simulink model "modele5vBhrol"  (R2024a)
settings: Solver=VariableStepAuto  StartTime=0.0  StopTime=120  RelTol=1e-9
values from neighbouring files (symbols this model uses):
  A_L = 1    [etablissement_variables.m]
  A_S = 3    [etablissement_variables.m]
  C_x = 0.2    [etablissement_variables.m]
  Cte_1 = 10    [etablissement_variables.m]
  Cte_2 = 1.9    [etablissement_variables.m]
  Cte_3 = 1    [etablissement_variables.m]
  Cte_4 = 0.97    [etablissement_variables.m]
  d_f = 1    [etablissement_variables.m]
  d_r = 1    [etablissement_variables.m]
  EPSILON = 1e-9    (= 1e-09)    [etablissement_variables.m]
  f = 0.1    [etablissement_variables.m]
  g = 9.81    [etablissement_variables.m]
  h = 0.4    [etablissement_variables.m]
  Iz = 500    [etablissement_variables.m]
  J = mr/2*R.^2    [etablissement_variables.m]
  L = l_r+l_f    (= 2.9)    [etablissement_variables.m]
  l_f = 1.7    [etablissement_variables.m]
  l_r = 1.2    [etablissement_variables.m]
  M = 400    [etablissement_variables.m]
  R = [0.52 0.52 0.52 0.52]    [etablissement_variables.m]
  rho = 1    [etablissement_variables.m]
undefined symbols (not defined in the file or in its folder): calcul_adherence, calcul_delta, calcul_forceaero, calcul_forces, calcul_lambda, calcul_moteur, calcul_N, calcul_normevitesseroue, calcul_omega, calcul_omegaackermann, calcul_retourvitesse, calcul_rotaroute, calcul_slipangle, calcul_vitessesroues, check_zeros_1, check_zeros_8, eqpfd, projection, reconstructionPi
libraries: simulink x5, slpidlib x2, embmathops x1
settings Model: Creator=TP-EEA  LastModifiedBy=TP-EEA

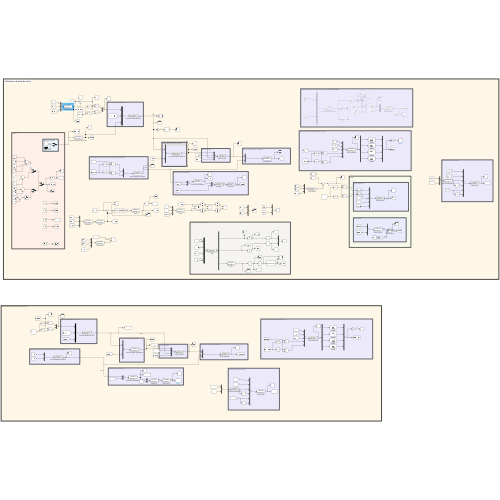
[thumbnail: Simulink's stored preview of the top-level diagram]
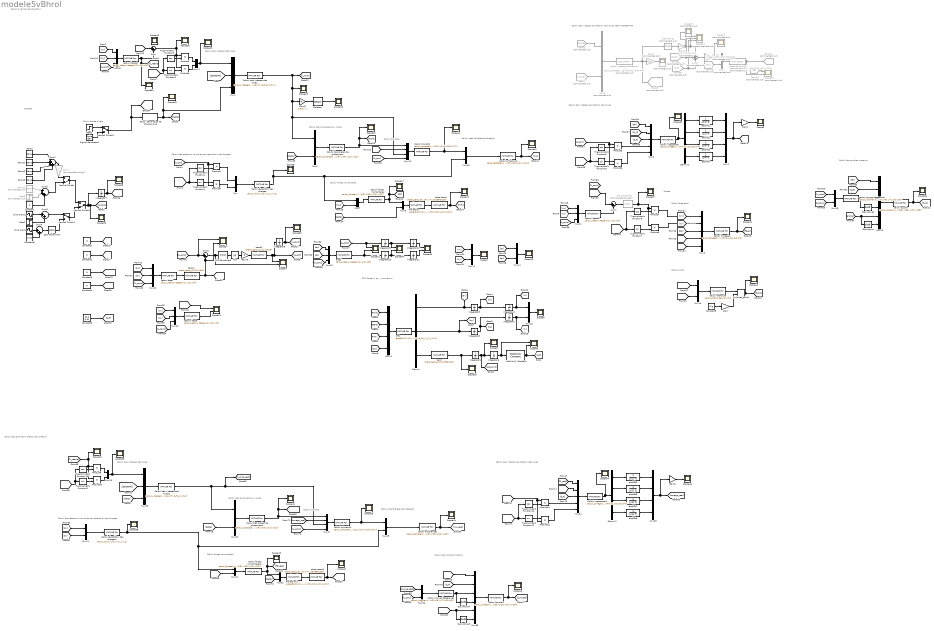
== system modele5vBhrol ==
  note: Calcul des grandeurs réelles (sans retour)
  note: Calcul avec boucle de retour
  note: Calcul des vitesses des roues
  note: Entrées
  note: Choix entrée angle
  note: Calcul des vitesses de rotation des roues
  note: PFD (forces x et y, moment z)
  note: Calcul poids
  note: Calcul des slip-angle aux roues
  note: Calcul coef adhérence (Pacejka)
  note: Calcul slip-ratio
  note: Calcul des réactions normales par répartition des charges
  note: Calcul forces horizontales
  note: Forces
  note: Calcul force aéro
  note: Calcul des vitesses de rotation des roues TEST ACKERMANN
  note: Calcul des réactions normales par répartition des charges
  note: Calcul des couples moteurs
  note: Calcul des vitesses des roues
  note: Calcul slip-ratio
  note: Calcul coef adhérence (Pacejka)
  note: Calcul des slip-angle aux roues
  note: Calcul forces horizontales
  note: Calcul des vitesses de rotation des roues
  note: Calcul des couples moteurs
  Abs : Abs  SaturateOnIntegerOverflow=off
  Calcul adhérence : MATLABFcn  MATLABFcn=calcul_adherence(u(1),u(2),u(3),u(4),u(5),u(6),u(7),u(8),Cte_1,Cte_2,Cte_3,Cte_4,u(9),u(10),u(11),u(12))  OutputDimensions=4*2
  Calcul adhérence1 : MATLABFcn  MATLABFcn=calcul_adherence(u(1),u(2),u(3),u(4),u(5),u(6),u(7),u(8),Cte_1,Cte_2,Cte_3,Cte_4,u(9),u(10),u(11),u(12))  OutputDimensions=4*2
  Calcul des angles de chaque roue : MATLABFcn  MATLABFcn=calcul_delta(u,L,d_f)  OutputDimensions=4
  Calcul des angles de glissement : MATLABFcn  MATLABFcn=calcul_slipangle(u(1),u(2),u(3),u(4),u(5),u(6),u(7),u(8),u(9),u(10),u(11),u(12))  OutputDimensions=4
  Calcul des angles de glissement1 : MATLABFcn  MATLABFcn=calcul_slipangle(u(1),u(2),u(3),u(4),u(5),u(6),u(7),u(8),u(9),u(10),u(11),u(12))  OutputDimensions=4
  Calcul des vitesses des roues : MATLABFcn  MATLABFcn=calcul_vitessesroues(u(1),u(2),u(3),u(4),u(5),u(6),u(7),d_f,d_r,l_f,l_r)  OutputDimensions=8
  Calcul des vitesses des roues1 : MATLABFcn  MATLABFcn=calcul_vitessesroues(u(1),u(2),u(3),u(4),u(5),u(6),u(7),d_f,d_r,l_f,l_r)  OutputDimensions=8
  Calcul forceaéro : MATLABFcn  MATLABFcn=calcul_forceaero(u(1),u(2),u(3),u(4),u(5),C_x,A_L,A_S,rho)  OutputDimensions=2
  Calcul forces horizontales : MATLABFcn  MATLABFcn=calcul_forces(u(1),u(2),u(3),u(4),u(5),u(6),u(7),u(8),u(9),u(10),u(11),u(12))  OutputDimensions=4*2
  Calcul forces horizontales1 : MATLABFcn  MATLABFcn=calcul_forces(u(1),u(2),u(3),u(4),u(5),u(6),u(7),u(8),u(9),u(10),u(11),u(12))  OutputDimensions=4*2
  Calcul rotaroute : MATLABFcn  MATLABFcn=calcul_rotaroute(u(1),u(2))  OutputDimensions=[3 3]  Output1D=off
  Calcul répartition des charges : MATLABFcn  MATLABFcn=calcul_N(u(1),u(2),M,L,l_r,h,g)  OutputDimensions=4
  Calcul répartition des charges1 : MATLABFcn  MATLABFcn=calcul_N(u(1),u(2),M,L,l_r,h,g)  OutputDimensions=4
  Calcul slip-ratio : MATLABFcn  MATLABFcn=calcul_lambda(u(1),u(2),u(3),u(4),R(1),R(2),R(3),R(4),u(5),u(6),u(7),u(8),u(9),u(11),u(13),u(15),u(10),u(12),u(14),u(16),u(17))  OutputDimensions=4*2
  Calcul slip-ratio1 : MATLABFcn  MATLABFcn=calcul_lambda(u(1),u(2),u(3),u(4),R(1),R(2),R(3),R(4),u(5),u(6),u(7),u(8),u(9),u(11),u(13),u(15),u(10),u(12),u(14),u(16),u(17))  OutputDimensions=4*2
  Calcul vitesserota : MATLABFcn  MATLABFcn=calcul_omega(u(1),u(2),u(3),u(4),u(5),u(6),u(7),u(8),u(9),u(10),u(11),u(12),u(13),u(14),u(15),u(16),u(17),u(18),R(1),R(2),R(3),R(4),J(1),J(2),J(3),J(4))  OutputDimensions=4
  Calcul vitesserota1 : MATLABFcn  MATLABFcn=calcul_omega(u(1),u(2),u(3),u(4),u(5),u(6),u(7),u(8),u(9),u(10),u(11),u(12),u(13),u(14),u(15),u(16),u(17),u(18),R(1),R(2),R(3),R(4),J(1),J(2),J(3),J(4))  OutputDimensions=4
  Calcul vitesserotaAckermann : MATLABFcn  Commented=on  MATLABFcn=calcul_omegaackermann(u(1),u(2),u(3),u(4),u(5),u(6),u(7),u(8),u(9),u(10),u(11),u(12),R(1),R(2),R(3),R(4))  OutputDimensions=4
  Constant{,1..4} (5 alike) : Constant  Value=0
  Constant5 : Constant  Value=M*g  VectorParams1D=off
  Constant6 : Constant  Value=1.01
  Constant8 : Constant  Value=[0 0 0 0]
  Demux : Demux  Outputs=3
  Demux1 : Demux
  Demux2 : Demux
  Derivative{,2..4} (4 alike) : Derivative
  Derivative1 : Derivative  Commented=on
  From12 : From  Commented=on  GotoTag=V_roue
  From36 : From  Commented=on  GotoTag=C_M
  From39 : From  Commented=on  GotoTag=C_F
  From43 : From  Commented=on  GotoTag=FP
  From46 : From  Commented=on  GotoTag=mu
  From6 : From  Commented=on  GotoTag=alpha
  Gain : Gain  Gain=[0 0 1]'
  Gain1 : Gain  Gain=30/pi
  Gain2 : Gain  Commented=on  Gain=[J(1) J(2) J(3) J(4)]
  Gain3 : Gain  Commented=on  Gain=-1./[R(1) R(2) R(3) R(4)]
  Gain4 : Gain  Commented=on  Gain=30/pi
  Gain5 : Gain  Gain=1/R(1)  Multiplication=Matrix(K*u)
  Gain6 : Gain  Gain=30/pi
  Gain7 : Gain  Commented=through  Gain=-1  Multiplication=Matrix(K*u)
  Gain8 : Gain  Gain=-1
  Goto24 : Goto  Commented=on  GotoTag=Fi_comp
  Goto25 : Goto  Commented=on  GotoTag=omega_comp
  Integrator{1..12} (12 alike) : Integrator
  Manual Switch : ManualSwitch  CurrentSetting=0
  Manual Switch1 : ManualSwitch
  Manual Switch2 : ManualSwitch
  Manual Switch3 : ManualSwitch  CurrentSetting=0
  Modulo by Constant : embmathops/Modulo by Constant  Denominator=2*pi  SimulateUsing=Code generation
      settings: LibrarySourceBlock=embeddedMathLib/Modulo by Constant
  Mux{,6..8,10,12..14,16..17,24..26,29..32,36} (18 alike) : Mux  Inputs=2
  Mux{1,11,15,27,33} (5 alike) : Mux
  Mux{2,18..22,28} (7 alike) : Mux  Inputs=3
  Mux23 : Mux  Inputs=6
  Mux3 : Mux  Commented=on  Inputs=2
  Mux34 : Mux  Inputs=5
  Mux35 : Mux  Inputs=6
  Mux4 : Mux  Commented=on  Inputs=2
  Mux5 : Mux  Inputs=5
  Mux9 : Mux  Inputs=5
  PFD : MATLABFcn  MATLABFcn=eqpfd(u(1),u(2),u(4),u(5),u(6),u(7),u(8),u(9),u(10),u(11),u(12),u(13),u(14),d_f,d_r,l_f,l_r,M,Iz)  OutputDimensions=3
  PID Controller1 : slpidlib/PID Controller  Commented=through  Controller=PID  Form=Parallel  TimeDomain=Continuous-time  UseExternalTs=off  SampleTime=-1  IntegratorMethod=Forward Euler  FilterMethod=Forward Euler  ControllerParametersSource=internal  P=5  I=1  UseKiTs=off  D=10  UseExternalDerivativeSource=off  N=100  UseFilter=on  TunerSelectOption=Transfer Function Based (PID Tuner App)  InitialConditionSource=internal  InitialConditionForIntegrator=0  InitialConditionForFilter=0  DifferentiatorICPrevScaledInput=0  ExternalReset=none  TrackingMode=off  Kt=1  LimitOutput=off  SatLimitsSource=internal  UpperSaturationLimit=inf  LowerSaturationLimit=-inf  LinearizeAsGain=on  AntiWindupMode=none  Kb=1  LimitIntegrator=off  UpperIntegratorSaturationLimit=inf  LowerIntegratorSaturationLimit=-inf  POutMin=[]  POutMax=[]  IOutMin=[]  IOutMax=[]  DOutMin=[]  DOutMax=[]  NOutMin=[]  NOutMax=[]  SumOutMin=[]  SumOutMax=[]  SaturationOutMin=[]  SaturationOutMax=[]  PParamMin=[]  PParamMax=[]  IParamMin=[]  IParamMax=[]  DParamMin=[]  DParamMax=[]  NParamMin=[]  NParamMax=[]  KbParamMin=[]  KbParamMax=[]  KtParamMin=[]  KtParamMax=[]  KbOutMin=[]  KbOutMax=[]  KtOutMin=[]  KtOutMax=[]  IntegratorOutMin=[]  IntegratorOutMax=[]  FilterOutMin=[]  FilterOutMax=[]  SumI1OutMin=[]  SumI1OutMax=[]  SumI2OutMin=[]  SumI2OutMax=[]  SumI3OutMin=[]  SumI3OutMax=[]  SumI4OutMin=[]  SumI4OutMax=[]  SumDOutMin=[]  SumDOutMax=[]  DifferentiatorOutMin=[]  DifferentiatorOutMax=[]  FilterDiffOutCoefMin=[]  FilterDiffOutCoefMax=[]  ReciprocalOutMin=[]  ReciprocalOutMax=[]  SumDenOutMin=[]  SumDenOutMax=[]  SumNumOutMin=[]  SumNumOutMax=[]  DivideOutMin=[]  DivideOutMax=[]  UdiffTsProdOutMin=[]  UdiffTsProdOutMax=[]  NTsProdOutMin=[]  NTsProdOutMax=[]  UintegralTsProdOutMin=[]  UintegralTsProdOutMax=[]  UngainTsProdOutMin=[]  UngainTsProdOutMax=[]  ClampingZeroOutDataTypeStr=Inherit: Inherit via back propagation  ClampingZeroOutMin=[]  ClampingZeroOutMax=[]  FilterDenConstantOutDataTypeStr=Inherit: Inherit via back propagation  FilterDenConstantOutMin=[]  FilterDenConstantOutMax=[]  PCopyOutDataTypeStr=Inherit: Inherit via back propagation  PCopyOutMin=[]  PCopyOutMax=[]  NCopyOutDataTypeStr=Inherit: Inherit via back propagation  NCopyOutMin=[]  NCopyOutMax=[]  IntegratorContinuousStateAttributes=''  IntegratorStateMustResolveToSignalObject=off  IntegratorRTWStateStorageClass=Auto  FilterContinuousStateAttributes=''  FilterStateMustResolveToSignalObject=off  FilterRTWStateStorageClass=Auto  ParallelPVariant=InternalParameters  IdealPVariant=Disabled  IVariant=InternalParameters  DVariant=InternalParameters  IntegratorVariant=Continuous  SatVariant=Disabled  AWVariant=Passthrough  PCopyVariant=Disabled  TRVariant=Disabled  FdbkBlocksVariant=Forward  IdealPFdbkVariant=Disabled  SatFdbkVariant=Disabled  DerivativeFilterVariant=ContFilter  NVariant=InternalParameters  NCopyVariant=Disabled  FilterICVariant=InternalICsFilter  IntegratorICVariant=InternalICs  ExternalResetVariant=Disabled  TRSumVariant=Passthrough  SumFdbkVariant=Disabled  SumVariant=Sum_PID  TsampFilterVariant=InternalTs  TsampNgainVariant=Passthrough  TsampIntegralVariant=Disabled_SignalSpec  ExternalSaturationOutDataTypeStr=Inherit: Same as second input  DerivativeSourceVariant=ErrorSignal
  PID Controller3 : slpidlib/PID Controller  Controller=PID  Form=Ideal  TimeDomain=Continuous-time  UseExternalTs=off  SampleTime=-1  IntegratorMethod=Forward Euler  FilterMethod=Forward Euler  ControllerParametersSource=internal  P=1  I=100  UseKiTs=off  D=0  UseExternalDerivativeSource=off  N=300  UseFilter=on  TunerSelectOption=Frequency Response Based  InitialConditionSource=internal  InitialConditionForIntegrator=0  InitialConditionForFilter=0  DifferentiatorICPrevScaledInput=0  ExternalReset=none  TrackingMode=off  Kt=1  LimitOutput=off  SatLimitsSource=internal  UpperSaturationLimit=inf  LowerSaturationLimit=-inf  LinearizeAsGain=on  AntiWindupMode=none  Kb=1  LimitIntegrator=off  UpperIntegratorSaturationLimit=inf  LowerIntegratorSaturationLimit=-inf  POutMin=[]  POutMax=[]  IOutMin=[]  IOutMax=[]  DOutMin=[]  DOutMax=[]  NOutMin=[]  NOutMax=[]  SumOutMin=[]  SumOutMax=[]  SaturationOutMin=[]  SaturationOutMax=[]  PParamMin=[]  PParamMax=[]  IParamMin=[]  IParamMax=[]  DParamMin=[]  DParamMax=[]  NParamMin=[]  NParamMax=[]  KbParamMin=[]  KbParamMax=[]  KtParamMin=[]  KtParamMax=[]  KbOutMin=[]  KbOutMax=[]  KtOutMin=[]  KtOutMax=[]  IntegratorOutMin=[]  IntegratorOutMax=[]  FilterOutMin=[]  FilterOutMax=[]  SumI1OutMin=[]  SumI1OutMax=[]  SumI2OutMin=[]  SumI2OutMax=[]  SumI3OutMin=[]  SumI3OutMax=[]  SumI4OutMin=[]  SumI4OutMax=[]  SumDOutMin=[]  SumDOutMax=[]  DifferentiatorOutMin=[]  DifferentiatorOutMax=[]  FilterDiffOutCoefMin=[]  FilterDiffOutCoefMax=[]  ReciprocalOutMin=[]  ReciprocalOutMax=[]  SumDenOutMin=[]  SumDenOutMax=[]  SumNumOutMin=[]  SumNumOutMax=[]  DivideOutMin=[]  DivideOutMax=[]  UdiffTsProdOutMin=[]  UdiffTsProdOutMax=[]  NTsProdOutMin=[]  NTsProdOutMax=[]  UintegralTsProdOutMin=[]  UintegralTsProdOutMax=[]  UngainTsProdOutMin=[]  UngainTsProdOutMax=[]  ClampingZeroOutDataTypeStr=Inherit: Inherit via back propagation  ClampingZeroOutMin=[]  ClampingZeroOutMax=[]  FilterDenConstantOutDataTypeStr=Inherit: Inherit via back propagation  FilterDenConstantOutMin=[]  FilterDenConstantOutMax=[]  PCopyOutDataTypeStr=Inherit: Inherit via back propagation  PCopyOutMin=[]  PCopyOutMax=[]  NCopyOutDataTypeStr=Inherit: Inherit via back propagation  NCopyOutMin=[]  NCopyOutMax=[]  IntegratorContinuousStateAttributes=''  IntegratorStateMustResolveToSignalObject=off  IntegratorRTWStateStorageClass=Auto  FilterContinuousStateAttributes=''  FilterStateMustResolveToSignalObject=off  FilterRTWStateStorageClass=Auto  ParallelPVariant=Passthrough  IdealPVariant=InternalParameters  IVariant=InternalParameters  DVariant=InternalParameters  IntegratorVariant=Continuous  SatVariant=Disabled  AWVariant=Passthrough  PCopyVariant=Disabled  TRVariant=Disabled  FdbkBlocksVariant=Forward  IdealPFdbkVariant=Disabled  SatFdbkVariant=Disabled  DerivativeFilterVariant=ContFilter  NVariant=InternalParameters  NCopyVariant=Disabled  FilterICVariant=InternalICsFilter  IntegratorICVariant=InternalICs  ExternalResetVariant=Disabled  TRSumVariant=Passthrough  SumFdbkVariant=Disabled  SumVariant=Sum_PID  TsampFilterVariant=InternalTs  TsampNgainVariant=Passthrough  TsampIntegralVariant=Disabled_SignalSpec  ExternalSaturationOutDataTypeStr=Inherit: Same as second input  DerivativeSourceVariant=ErrorSignal
  Product{1..12} (12 alike) : Product
  Projection : MATLABFcn  MATLABFcn=projection(u(1),u(2),u(3),u(4),u(5),u(6),u(7),u(8),u(9),u(10),u(11),u(12))  OutputDimensions=8
  Projection1 : MATLABFcn  MATLABFcn=projection(u(1),u(2),u(3),u(4),u(5),u(6),u(7),u(8),u(9),u(10),u(11),u(12))  OutputDimensions=8
  Ramp : simulink/Sources/Ramp  slope=1  start=0  InitialOutput=0
  Ramp1 : simulink/Sources/Ramp  slope=-1  start=3  InitialOutput=0
  Ramp2 : simulink/Sources/Ramp  slope=-1  start=7  InitialOutput=0
  Ramp3 : simulink/Sources/Ramp  slope=1  start=9  InitialOutput=0
  Ramp4 : simulink/Sources/Ramp  Commented=on  slope=-1  start=0  InitialOutput=0
  ReconstructionPi : MATLABFcn  Commented=on  MATLABFcn=reconstructionPi(u(1),u(2),u(3),u(4),u(5),u(6),u(7),u(8),u(9),u(10),u(11),u(12))  OutputDimensions=8
  Scope1 : Scope  Commented=on
  Scope{2..3,6..8,10..20,25..26,28..30,32..33,36..50} (38 alike) : Scope
  Scope{4,9,21..22,27,34..35} (7 alike) : Scope  NumInputPorts=2
  Scope23 : Scope  Commented=on  NumInputPorts=2
  Scope24 : Scope  Commented=on  NumInputPorts=3
  Scope31 : Scope  Commented=on
  Scope5 : Scope  Commented=on
  Selector : Selector  InputPortWidth=8  IndexOptions=Index vector (dialog)  Indices=[1,3,5,7]  OutputSizes=1
  Signal Generator2 : SignalGenerator  Amplitude=0.2  Frequency=0.1  Units=rad/sec
  Sine Wave : Sin  Frequency=0.1  SampleTime=0
  Sine Wave1 : Sin  SampleTime=0
  Step1 : Step  Time=0  After=0  SampleTime=0
  Step2 : Step  Time=0  After=0  SampleTime=0
  Step3 : Step  Commented=on  Time=0  SampleTime=0
  Sum : Sum  Inputs=|+-
  Sum1 : Sum  Inputs=|++++
  Sum2 : Sum  Commented=on  Inputs=+-+
  Sum3 : Sum  Inputs=|+-
  Sum4 : Sum  Inputs=|++
  Sum5 : Sum  Inputs=|++
  Sum6 : Sum  Inputs=|+++
  Sum7 : Sum  Inputs=|+-
  Trigonometric Function{1..2,5,7,9,11} (6 alike) : Trigonometry
  Trigonometric Function{3..4,6,8,10,12} (6 alike) : Trigonometry  Operator=cos
  Zero-Order Hold : ZeroOrderHold  SampleTime=3
  accel : MATLABFcn  MATLABFcn=calcul_retourvitesse(u(1),u(2),u(3))  OutputDimensions=1
  calcul couple : MATLABFcn  MATLABFcn=calcul_moteur(u(1),u(2),u(3),u(4),u(5),u(6),u(7),u(8),u(9),u(10),u(11),u(12),R(1),R(2),R(3),R(4),J(1),J(2),J(3),J(4),u(13),u(14),u(15),u(16),u(17),u(18),u(19),u(20),u(21),u(22),u(23),u(24),u(25),u(26),u(27),u(28))  OutputDimensions=4
  calcul couple1 : MATLABFcn  MATLABFcn=calcul_moteur(u(1),u(2),u(3),u(4),u(5),u(6),u(7),u(8),u(9),u(10),u(11),u(12),R(1),R(2),R(3),R(4),J(1),J(2),J(3),J(4),u(13),u(14),u(15),u(16),u(17),u(18),u(19),u(20),u(21),u(22),u(23),u(24),u(25),u(26),u(27),u(28))  OutputDimensions=4
  calcul normevitesseroue : MATLABFcn  MATLABFcn=calcul_normevitesseroue(u(1),u(2),u(3),u(4),u(5),u(6),u(7),u(8),u(9))  OutputDimensions=4
  calcul normevitesseroue1 : MATLABFcn  MATLABFcn=calcul_normevitesseroue(u(1),u(2),u(3),u(4),u(5),u(6),u(7),u(8),u(9))  OutputDimensions=4
  check zeros : MATLABFcn  MATLABFcn=check_zeros_8(u(1),u(2),u(3),u(4),u(5),u(6),u(7),u(8),EPSILON)  OutputDimensions=8
  check zeros1 : MATLABFcn  MATLABFcn=check_zeros_8(u(1),u(2),u(3),u(4),u(5),u(6),u(7),u(8),EPSILON)  OutputDimensions=8
  eqdiffz1 : TransferFcn  Denominator=[J(1) f]
  eqdiffz2 : TransferFcn  Denominator=[J(2) f]
  eqdiffz3 : TransferFcn  Denominator=[J(3) f]
  eqdiffz4 : TransferFcn  Denominator=[J(4) f]
  eqdiffz5 : TransferFcn  Denominator=[J(1) f]
  eqdiffz6 : TransferFcn  Denominator=[J(2) f]
  eqdiffz7 : TransferFcn  Denominator=[J(3) f]
  eqdiffz8 : TransferFcn  Denominator=[J(4) f]
  multmat_poids : Product  Multiplication=Matrix(*)
  retour accel : MATLABFcn  MATLABFcn=calcul_retourvitesse(u(1),u(2),u(3))  OutputDimensions=1
  retourvitesse : MATLABFcn  MATLABFcn=calcul_retourvitesse(u(1),u(2),u(3))  OutputDimensions=1
  retourvitesse1 : MATLABFcn  MATLABFcn=calcul_retourvitesse(u(1),u(2),u(3))  OutputDimensions=1
  retourvitesse2 : MATLABFcn  MATLABFcn=calcul_retourvitesse(u(1),u(2),u(3))  OutputDimensions=1
  zeros : MATLABFcn  MATLABFcn=check_zeros_1(u(1),EPSILON)
  zeros1 : MATLABFcn  MATLABFcn=check_zeros_1(u(1),1e-9)
  zeros2 : MATLABFcn  MATLABFcn=check_zeros_1(u(1),1e-15)
  wires:
  accel/1 -> Integrator10/1, Scope21/2
  Calcul des angles de glissement/1 -> [alpha], Scope13/1, Mux15/1
  Mux17/1 -> Scope20/1, Mux2/1
  [Vventy] -> Mux9/5
  [ay] -> Mux22/2
  [ax] -> Mux22/1
  Mux9/1 -> Calcul forceaéro/1
  Mux2/1 -> Calcul des vitesses des roues/1
  Calcul adhérence/1 -> Scope16/1, [mu]
  [A_cons] -> Scope27/1, Sum3/1
  Mux22/1 -> retour accel/1
  [thetaroute] -> Mux10/1
  [Vx] -> Mux20/1
  eqdiffz4/1 -> Mux1/4
  [Faero] -> Mux11/2
  retourvitesse/1 -> Scope22/2  "V"
  [ax] -> Mux19/1
  Mux11/1 -> PFD/1
  [A_cons] -> Integrator9/1, Scope21/1
  [Poids] -> Mux11/1
  Manual Switch2/1 -> [delta_com], Calcul des angles de chaque roue/1
  Trigonometric Function3/1 -> Product2/2
  Product2/1 -> Mux17/1
  Projection/1 -> check zeros/1  "FxFy"
  Trigonometric Function2/1 -> Product3/2
  [A_corr] -> Mux15/4
  PFD/1 -> Demux/1
  Mux8/1 -> Projection/1
  Constant5/1 -> Gain/1
  Mux6/1 -> Calcul des angles de glissement/1
  Integrator2/1 -> Mux13/2, [y]
  Mux7/1 -> Calcul forces horizontales/1
  multmat_poids/1 -> Scope11/1, [Poids]  "P"
  Product3/1 -> Mux17/2
  Mux10/1 -> Calcul rotaroute/1
  Calcul forceaéro/1 -> Scope10/1, [Faero]  "forceaéro"
  Integrator1/1 -> Scope8/1, Integrator6/1, [psipoint]
  Mux15/1 -> Calcul slip-ratio/1
  [FxFy] -> Mux11/3
  [delta_com] -> Trigonometric Function3/1, Trigonometric Function2/1
  Gain/1 -> multmat_poids/2
  Mux20/1 -> retourvitesse/1
  [mu] -> Mux7/2
  Mux14/1 -> Scope15/1
  [psipoint] -> Mux2/2
  Integrator4/1 -> Mux13/1, [x]
  [Vventx] -> Mux9/4
  [psi] -> Mux9/3
  [ax] -> Mux14/1
  [ay] -> Mux14/2
  Mux12/1 -> Scope7/1
  Integrator5/1 -> Integrator4/1, [Vx]
  [phiroute] -> Mux10/2
  Integrator6/1 -> Modulo by Constant/1, Scope9/1
  [Vx] -> Mux12/1
  Mux13/1 -> Scope3/1
  Signal Generator2/1 -> Manual Switch2/2  "delta*"
  eqdiffz3/1 -> Mux1/3
  calcul couple/1 -> Scope36/1, [C_M]
  [Vy] -> Mux12/2
  Step1/1 -> Manual Switch2/1  "delta*"
  Calcul rotaroute/1 -> multmat_poids/1
  Constant1/1 -> [Vventx]
  Calcul des angles de chaque roue/1 -> [delta], Mux2/3, Scope18/1
  Calcul répartition des charges/1 -> Mux7/1, Mux16/2, Scope6/1  "N_cons"
  Constant4/1 -> [phiroute]
  Constant2/1 -> [Vventy]
  Integrator3/1 -> Integrator2/1, [Vy]
  Demux1/4 -> eqdiffz4/1
  Constant8/1 -> [C_F]
  eqdiffz2/1 -> Mux1/2
  [C_M] -> Mux5/2
  Mux19/1 -> accel/1
  Mux5/1 -> Calcul vitesserota/1
  Calcul vitesserota/1 -> Scope32/1, Demux1/1
  [delta] -> Mux8/2
  retour accel/1 -> zeros1/1  "A_ret"
  Mux1/1 -> Gain1/1, [omega]
  [C_F] -> Mux5/3
  eqdiffz1/1 -> Mux1/1
  Constant3/1 -> [thetaroute]
  Demux1/3 -> eqdiffz3/1
  Demux1/2 -> eqdiffz2/1
  Demux1/1 -> eqdiffz1/1
  Product4/1 -> Mux/2
  [ay] -> Mux19/2
  [Vy] -> Mux20/2
  Modulo by Constant/1 -> [psi], Scope9/2
  Manual Switch3/1 -> Integrator7/1, Scope33/1, [A_cons]
  Manual Switch/1 -> Manual Switch3/1
  Manual Switch1/1 -> Manual Switch3/2
  Zero-Order Hold/1 -> Manual Switch1/2
  Gain1/1 -> Scope2/1
  Sum1/1 -> Gain7/1
  From12/1 -> Mux3/2
  Mux3/1 -> Calcul vitesserotaAckermann/1
  Calcul vitesserotaAckermann/1 -> Gain4/1, Derivative1/1, Goto25/1
  Derivative1/1 -> Gain2/1
  Gain2/1 -> Scope31/1, Scope24/1, Sum2/1
  From36/1 -> Scope24/2, Sum2/2
  From39/1 -> Scope24/3, Sum2/3
  Sum2/1 -> Gain3/1
  From43/1 -> Scope23/1
  [omega] -> Mux15/2
  From46/1 -> Mux4/2
  Gain3/1 -> Scope1/1, Mux4/1
  Mux4/1 -> ReconstructionPi/1
  ReconstructionPi/1 -> Goto24/1, Scope23/2
  [FP] -> Mux5/1
  [V_voulue] -> Scope22/1  "Vvoulue"
  zeros/1 -> Scope29/1, Integrator1/1
  Gain4/1 -> Scope5/1
  Integrator8/1 -> Scope30/1, [V_cons]
  PID Controller3/1 -> Abs/1
  Gain5/1 -> Selector/1
  Selector/1 -> Scope25/1
  From6/1 -> Mux3/1
  [Vy] -> Mux18/2
  [Vx] -> Mux18/1
  [V_voulue] -> Sum/1
  retourvitesse2/1 -> Sum/2, Scope50/1, [V_reelle]  "V"
  Mux18/1 -> retourvitesse2/1
  [psi] -> Mux11/4
  [delta] -> Mux6/2
  Calcul forces horizontales/1 -> Scope17/1, [FP], Mux8/1
  Mux/1 -> Calcul répartition des charges/1
  Calcul des vitesses des roues/1 -> Gain5/1, Mux6/1, Mux15/3, Scope19/1, [V_roue]  "Vrcons"
  [FP] -> Mux23/1
  [C_F] -> Mux23/2
  Mux23/1 -> calcul couple/1
  check zeros/1 -> Scope12/1, [FxFy]  "FxFy"
  Sum/1 -> Scope26/1, Product3/1, Product2/1
  Ramp/1 -> Sum1/1
  Ramp1/1 -> Sum1/2
  Ramp2/1 -> Sum1/3
  Ramp3/1 -> Sum1/4
  Integrator7/1 -> [V_voulue], Scope28/1
  [delta_com] -> Trigonometric Function4/1, Trigonometric Function1/1
  Trigonometric Function1/1 -> Product4/1
  Product1/1 -> Mux/1
  Trigonometric Function4/1 -> Product1/2
  [A_corr] -> Product1/1, Product4/2
  Product5/1 -> Mux5/4
  [delta_com] -> Trigonometric Function6/1, Trigonometric Function5/1
  [A_corr] -> Product5/1, Product6/2
  Product6/1 -> Mux5/5
  Trigonometric Function6/1 -> Product5/2
  Trigonometric Function5/1 -> Product6/1
  Sine Wave/1 -> Sum4/1
  Sum4/1 -> Zero-Order Hold/1
  Constant6/1 -> Sum4/2
  Sum5/1 -> Manual Switch1/1
  Sine Wave1/1 -> Sum5/1
  Step2/1 -> Sum5/2
  Integrator9/1 -> Integrator12/1, Scope34/1
  Integrator12/1 -> Scope35/1
  Integrator11/1 -> Scope35/2
  Integrator10/1 -> Integrator11/1, Scope34/2
  Sum6/1 -> Manual Switch/2
  Step3/1 -> Sum6/2
  Mux21/1 -> retourvitesse1/1
  PID Controller1/1 -> Scope37/1, Product8/1, Product7/1
  Product7/1 -> Mux9/1
  Sum7/1 -> PID Controller1/1
  Product8/1 -> Mux9/2
  [Vx] -> Mux21/1
  [delta_com] -> Trigonometric Function8/1, Trigonometric Function7/1
  Trigonometric Function7/1 -> Product8/2
  [V_voulue] -> Sum7/1
  [Vy] -> Mux21/2
  retourvitesse1/1 -> Sum7/2  "V"
  Trigonometric Function8/1 -> Product7/2
  [A_cons] -> Mux22/3
  [A_cons] -> Mux19/3
  [A_cons] -> Mux18/3
  [A_cons] -> Mux21/3
  [A_cons] -> Mux20/3
  Mux24/1 -> Calcul répartition des charges1/1
  [ay] -> Mux24/2
  [ax] -> Mux24/1
  Derivative/1 -> Mux23/6
  [alpha] -> Derivative/1, Mux23/5
  calcul normevitesseroue/1 -> Mux23/3, Derivative2/1
  Derivative2/1 -> Mux23/4
  Mux25/1 -> calcul normevitesseroue/1
  [V_roue] -> Mux25/1
  [A_cons] -> Mux25/2
  Ramp4/1 -> Sum6/1
  [V_reelle] -> Scope40/1, Product10/1, Product9/1
  [delta_com] -> Trigonometric Function10/1, Trigonometric Function9/1
  [psipoint] -> Mux28/2
  Trigonometric Function10/1 -> Product9/2
  Trigonometric Function9/1 -> Product10/2
  Product10/1 -> Mux26/2
  Mux26/1 -> Scope39/1, Mux28/1
  Mux28/1 -> Calcul des vitesses des roues1/1
  Product9/1 -> Mux26/1
  [delta] -> Mux28/3
  check zeros1/1 -> Scope41/1, [FxFy_reel]  "FxFy"
  Calcul adhérence1/1 -> Scope44/1, [mu_reel]
  Mux29/1 -> Calcul adhérence1/1
  Calcul forces horizontales1/1 -> Scope45/1, [FP_reel], Mux32/1
  Mux31/1 -> Calcul forces horizontales1/1
  [delta] -> Mux32/2
  [omega_reel] -> Mux27/2
  Calcul slip-ratio1/1 -> Mux29/1, Scope43/1
  Calcul répartition des charges1/1 -> Mux31/1, Mux29/2, Scope38/1  "N_cons"
  [A_cons] -> Mux27/4
  [mu_reel] -> Mux31/2
  Mux32/1 -> Projection1/1
  Mux27/1 -> Calcul slip-ratio1/1
  Mux30/1 -> Calcul des angles de glissement1/1
  [delta] -> Mux30/2
  Calcul des angles de glissement1/1 -> [alpha_reel], Scope42/1, Mux27/1
  Calcul des vitesses des roues1/1 -> Mux30/1, [V_roue_reel], Mux27/3  "Vrcons"
  Projection1/1 -> check zeros1/1  "FxFy"
  [FP_reel] -> Mux34/1
  Trigonometric Function12/1 -> Product11/2
  [A_reelle] -> Product11/1, Product12/2
  Demux2/4 -> eqdiffz8/1
  Trigonometric Function11/1 -> Product12/1
  Demux2/2 -> eqdiffz6/1
  Product11/1 -> Mux34/4
  Demux2/3 -> eqdiffz7/1
  eqdiffz6/1 -> Mux33/2
  eqdiffz5/1 -> Mux33/1
  Gain6/1 -> Scope46/1
  Calcul vitesserota1/1 -> Scope47/1, Demux2/1
  Mux33/1 -> Gain6/1, [omega_reel]
  [delta_com] -> Trigonometric Function12/1, Trigonometric Function11/1
  Mux34/1 -> Calcul vitesserota1/1
  Product12/1 -> Mux34/5
  [C_M_reel] -> Mux34/2
  eqdiffz7/1 -> Mux33/3
  eqdiffz8/1 -> Mux33/4
  Demux2/1 -> eqdiffz5/1
  [C_F] -> Mux34/3
  [A_cons] -> Mux36/2
  Derivative4/1 -> Mux35/4
  Derivative3/1 -> Mux35/6
  calcul normevitesseroue1/1 -> Mux35/3, Derivative4/1
  Mux35/1 -> calcul couple1/1
  [C_F] -> Mux35/2
  [V_roue_reel] -> Mux36/1
  calcul couple1/1 -> Scope48/1, [C_M_reel]
  [alpha_reel] -> Derivative3/1, Mux35/5
  Mux36/1 -> calcul normevitesseroue1/1
  [FP_reel] -> Mux35/1
  Gain7/1 -> Manual Switch/1
  Sum3/1 -> Scope4/2, PID Controller3/1
  Gain8/1 -> zeros2/1
  Abs/1 -> Gain8/1
  Demux/3 -> zeros/1
  Demux/2 -> [ay], Integrator3/1
  Demux/1 -> [ax], Integrator5/1
  Calcul slip-ratio/1 -> Mux16/1, Scope14/1
  Mux16/1 -> Calcul adhérence/1
  Constant/1 -> Sum6/3
  zeros1/1 -> [A_reelle], Sum3/2, Scope27/2
  zeros2/1 -> Integrator8/1, [A_corr], Scope4/1
